simulink model "lab3cancel_dynamics"  (R2023b)
settings: Solver=VariableStepAuto  StartTime=0.0  StopTime=10.0  RelTol=1e-3
values from neighbouring files (symbols this model uses):
  par = [3, 2, 1, 0.6, 5.0, 5.0, 9.81]    [lab3init.m]
settings Model: Creator=rpl  LastModifiedBy=rpl

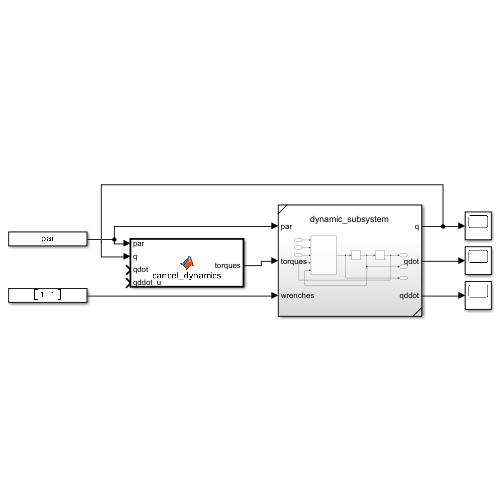
[thumbnail: Simulink's stored preview of the top-level diagram]
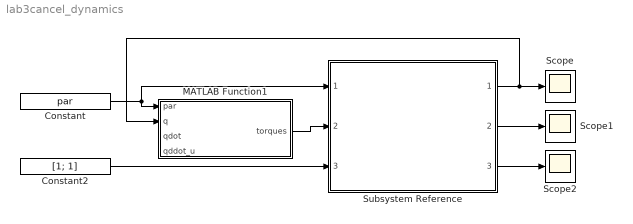
== system lab3cancel_dynamics ==
  Constant : Constant  Value=par
  Constant2 : Constant  Value=[1; 1]
  MATLAB Function1 : MATLAB Function  TreatAsAtomicUnit=on
  Scope : Scope
  Scope1 : Scope
  Scope2 : Scope
  Subsystem Reference : Subsystem  ReferencedSubsystem=dynamic_subsystem
  wires:
  Constant/1 -> MATLAB Function1/1(par), Subsystem Reference/1
  Constant2/1 -> Subsystem Reference/3
  MATLAB Function1/1(torques) -> Subsystem Reference/2
  Subsystem Reference/1 -> Scope/1, MATLAB Function1/2(q)
  Subsystem Reference/2 -> Scope1/1
  Subsystem Reference/3 -> Scope2/1

== matlab function lab3cancel_dynamics/MATLAB Function1 ==
  data: par input; q input; torques output; qdot input; qddot_u input
function torques = cancel_dynamics(par, q, qdot, qddot_u)

    m1 = par(1);
    m2 = par(2);
    l1 = par(3);
    l2 = par(4);
    b1 = par(5);
    b2 = par(6);
    g = par(7);

    % sines and cosines
    sq1 = sin(q(1));
    sq2 = sin(q(2));
    cq1 = cos(q(1));
    cq2 = cos(q(2));
    sq12 = sin(q(1)+q(2));
    cq12 = cos(q(1)+q(2));
    
    % Calculate M(1)
    Msim = m2*(l1*l2*cq2 + l2^2); % simetrical term
    M = [m1*l1^2+m2*(l1^2+2*l1*l2*cq2+l2^2), Msim;
         Msim, m2*l2^2];
         
    % Calculate C(q, qdot)*qdot
    Cqdot = [-m2*l1*l2*sq2*(2*qdot(1)*qdot(2)+qdot(2)^2);
              m2*l1*l2*qdot(1)^2*sq2];

    % Calculate Fb
    Fb = [b1, 0;
          0, b2];

    % Calculate g(q)
    gvec = [(m1+m2)*l1*g*cq1+m2*g*l2*cq12;
          m2*g*l2*cq12];

    % Control torque  to cancel the dynamic model
    % leave only desired joint acceleration (qddot_u)
    torque = M * qddot_u + Cqdot + Fb * qdot + gvec);
